simulink model "closed_loop"  (R2025b)
settings: Solver=VariableStepAuto  StartTime=0.0  StopTime=800  RelTol=1e-3
model workspace (MAT data in the model file):
  C_i = -12.5046
  J_i = -40.0148
  J_p = -143.4271
  alpha = 14.0311
  beta = 0.0025
  l_eff = 0.4303
  omega_n = 4.7745
settings Model: Creator=benricket  LastModifiedBy=choang

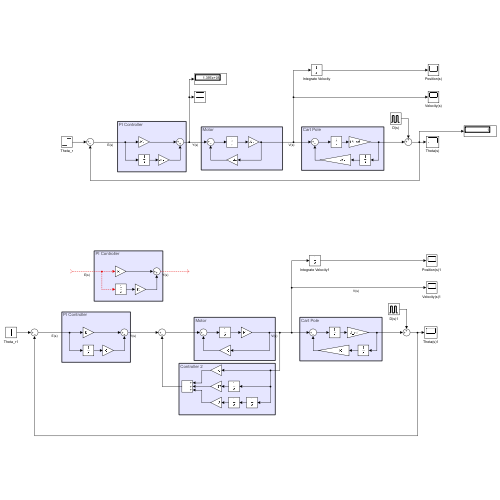
[thumbnail: Simulink's stored preview of the top-level diagram]
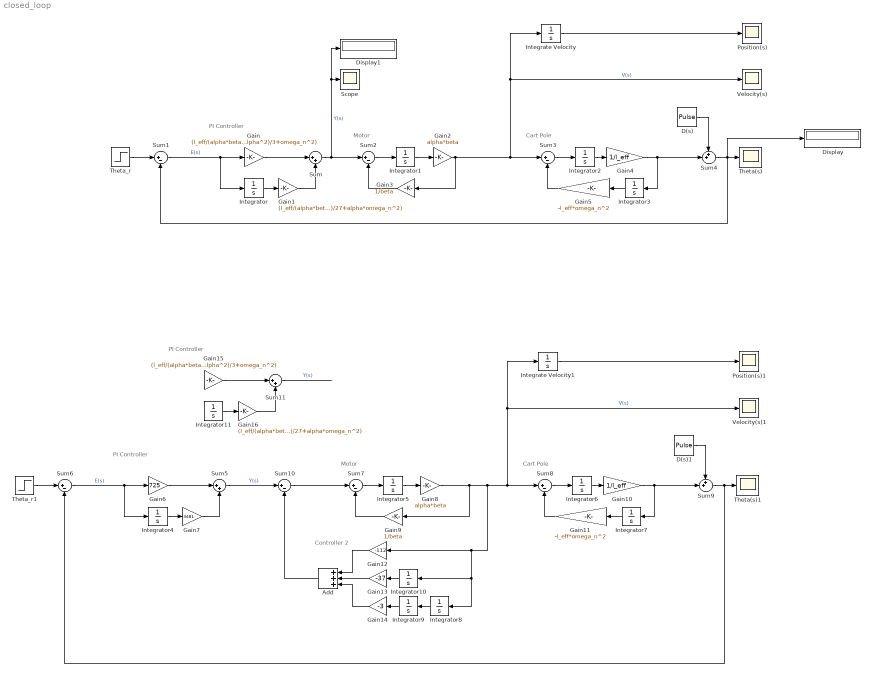
== system closed_loop ==
  note: Controller 2
  note: Cart Pole
  note: PI Controller
  note: Motor
  note: Cart Pole
  note: Motor
  note: PI Controller
  note: PI Controller
  Add : Sum  Inputs=+++
  D(s) : DiscretePulseGenerator  PulseType=Time based  Period=100  PulseWidth=0.1
  D(s)1 : DiscretePulseGenerator  PulseType=Time based  Amplitude=.5  Period=100  PulseWidth=0.1
  Display : Display
  Display1 : Display
  Gain : Gain  Gain=(l_eff/(alpha*beta))*((alpha^2)/3+omega_n^2)
  Gain1 : Gain  Gain=(l_eff/(alpha*beta))*((alpha^2)/27+alpha*omega_n^2)
  Gain10 : Gain  Gain=1/l_eff
  Gain11 : Gain  Gain=-l_eff*omega_n^2
  Gain12 : Gain  Gain=-112
  Gain13 : Gain  Gain=-37
  Gain14 : Gain  Gain=-3
  Gain15 : Gain  Gain=(l_eff/(alpha*beta))*((alpha^2)/3+omega_n^2)
  Gain16 : Gain  Gain=(l_eff/(alpha*beta))*((alpha^2)/27+alpha*omega_n^2)
  Gain2 : Gain  Gain=alpha*beta
  Gain3 : Gain  Gain=1/beta
  Gain4 : Gain  Gain=1/l_eff
  Gain5 : Gain  Gain=-l_eff*omega_n^2
  Gain6 : Gain  Gain=725
  Gain7 : Gain  Gain=3481
  Gain8 : Gain  Gain=alpha*beta
  Gain9 : Gain  Gain=1/beta
  Integrate Velocity : Integrator
  Integrate Velocity1 : Integrator
  Integrator{,1..11} (12 alike) : Integrator
  Position(s) : Scope
      settings: ActiveDisplayYMinimum=-1  ActiveDisplayYMaximum=1
  Position(s)1 : Scope
      settings: ActiveDisplayYMinimum=-0.66505541342204155  ActiveDisplayYMaximum=4.8750457784483494
  Scope : Scope
      settings: ActiveDisplayYMinimum=-1  ActiveDisplayYMaximum=1  DataLoggingVariableName=ScopeData4
  Sum : Sum  Inputs=|++
  Sum{1..3,6..8,10} (7 alike) : Sum  Inputs=|+-
  Sum11 : Sum  Inputs=|++
  Sum4 : Sum  Inputs=++|
  Sum5 : Sum  Inputs=|++
  Sum9 : Sum  Inputs=++|
  Theta(s) : Scope
      settings: ActiveDisplayYMinimum=-1  ActiveDisplayYMaximum=1
  Theta(s)1 : Scope
      settings: ActiveDisplayYMinimum=-0.49006642804831535  ActiveDisplayYMaximum=0.61000738089425721  DataLoggingVariableName=ScopeData2
  Theta_r : Step  After=0  SampleTime=0
  Theta_r1 : Step  After=0  SampleTime=0
  Velocity(s) : Scope
      settings: ActiveDisplayYMinimum=-1  ActiveDisplayYMaximum=1  DataLoggingVariableName=ScopeData2
  Velocity(s)1 : Scope
      settings: ActiveDisplayYMinimum=-1.3717213087884881  ActiveDisplayYMaximum=3.0576033522268311  DataLoggingVariableName=ScopeData3
  wires:
  Integrator/1 -> Gain1/1
  Gain/1 -> Sum/1
  Gain1/1 -> Sum/2
  Sum1/1 -> Integrator/1, Gain/1  "E(s)"
  Theta_r/1 -> Sum1/1
  Integrator1/1 -> Gain2/1
  Gain2/1 -> Gain3/1, Velocity(s)/1, Integrate Velocity/1, Sum3/1  "V(s)"
  Sum2/1 -> Integrator1/1
  Gain3/1 -> Sum2/2
  Sum/1 -> Display1/1, Scope/1, Sum2/1  "Y(s)"
  Sum3/1 -> Integrator2/1
  Integrator2/1 -> Gain4/1
  Gain4/1 -> Sum4/2, Integrator3/1
  Integrator3/1 -> Gain5/1
  Gain5/1 -> Sum3/2
  D(s)/1 -> Sum4/1
  Sum4/1 -> Theta(s)/1, Sum1/2, Display/1
  Integrate Velocity/1 -> Position(s)/1
  Integrator4/1 -> Gain7/1
  Gain10/1 -> Sum9/2, Integrator7/1
  Sum9/1 -> Theta(s)1/1, Sum6/2
  Integrator7/1 -> Gain11/1
  Sum6/1 -> Integrator4/1, Gain6/1  "E(s)"
  Gain9/1 -> Sum7/2
  Gain6/1 -> Sum5/1
  Gain11/1 -> Sum8/2
  Sum8/1 -> Integrator6/1
  Theta_r1/1 -> Sum6/1
  Gain7/1 -> Sum5/2
  Sum7/1 -> Integrator5/1
  Integrator5/1 -> Gain8/1
  Integrate Velocity1/1 -> Position(s)1/1
  Gain8/1 -> Velocity(s)1/1, Integrate Velocity1/1, Sum8/1, Integrator8/1, Integrator10/1, Gain12/1, Gain9/1  "V(s)"
  Integrator6/1 -> Gain10/1
  D(s)1/1 -> Sum9/1
  Sum5/1 -> Sum10/1  "Y(s)"
  Sum10/1 -> Sum7/1
  Integrator9/1 -> Gain14/1
  Integrator8/1 -> Integrator9/1
  Integrator10/1 -> Gain13/1
  Gain12/1 -> Add/1
  Gain13/1 -> Add/2
  Gain14/1 -> Add/3
  Add/1 -> Sum10/2
  Gain16/1 -> Sum11/2
  Gain15/1 -> Sum11/1
  Integrator11/1 -> Gain16/1
  Sum11/1 -> ?  "Y(s)"
  ? -> Integrator11/1, Gain15/1  "E(s)"
